simulink library "powerlib2"  (Simulink 6.0)
settings: Solver=ode45  SolverMode=SingleTasking  StartTime=0.0  StopTime=10.0  RelTol=1e-3
undefined symbols (not defined in the file or in its folder): com, ctrl1, Da, DiscIntNeverNeededParam, dtha, etat, FA, gcbh, Ha, Ka, Lm, Ls, powericonV2, q0, Rm, Rs, sel, st_a, st_b, st_c, sta, stb, stc, T1, T2, T3, T4
libraries: powerlib2 x55, simulink_extras x5, powerlib_extras x4, powerlib_modelsV2 x4, simulink x1
(part 4 of 6)

== system powerlib2/Power Electronics ==
  note: ____ D e v i c e s __________________________________________________
  note: ____ E x t r a s ____________________________________________________
  "  Extra Library " : Subsystem
      settings: OpenFcn=sys=sprintf('%s\n%s','powerlib_extras/Discrete ','Control Blocks');powerlib_extras([],[],[],'load');open_system(sys)
      mask Display: disp(['Discrete Control blocks'])
  "  Extra Library 1" : Subsystem
      settings: OpenFcn=sys=sprintf('%s\n%s','powerlib_extras/Control ','Blocks');powerlib_extras([],[],[],'load');open_system(sys)
      mask Display: disp(['Control blocks'])
  Detailed Thyristor : Subsystem  Tag=PoWeRsYsTeMbLoCk  LoadFcn=powericonV2('psblfblk',bdroot,'gotofrom','Load');  mask(Detailed Thyristor){Ron=1e-3, Lon=0, Vf=0.8, IL=0.1, Tq=100e-6, IC=0, Rs=10, Cs=4.7e-6, PSBOutputType=10}
      mask prompts: Ron "Resistance Ron (Ohms) :"; Lon "Inductance Lon (H) :"; Vf "Forward voltage Vf (V) :"; IL "Latching current Il (A) :"; Tq "Turn-off time Tq (s) :"; IC "Initial current Ic (A) :"; Rs "Snubber resistance Rs (Ohms) :"; Cs "Snubber capacitance Cs (F) :"; PSBOutputType "Output type [1=PSB  0=simulink output]"
      mask help:
      | Detailed model of Thyristor in parallel with a series RC snubber circuit. In on-state the Thyristor model  has an internal resistance (Ron) and inductance (Lon).  For most applications the internal inductance should be set to zero. In off-state the Detailed Thyristor  as an impedance.
      |
      | Best accuracy is achieved when Tq is larger than the simulation step size.
      mask init:
      | s=powericonV2('PowerSwitch',Rs,Cs);
      settings: CopyFcn=powericonV2('psblfblk',bdroot,'gotofrom','Copy');
      mask Help: web(psbhelp);
      mask Display: plot(-140,-140,140,140,2*[-30,-30,0,-30,-30,-55]+25,(2*[20,0,20,41,20,20]+8),[0,0]+25,(2*[0,40]+8),2*[37.5,0]+25,(2*[20,20]+8),2*[10,10,0]+25,(1*[-15,6,20]+12),s*[-65,-65,-20,-20,40,40,85,85,85,40,40,-20,-20],s*[48,-20,-20,-10,-10,-20,-20,48,-20,-20,-30,-30,-20])
  Diode : Subsystem  Tag=PoWeRsYsTeMbLoCk  LoadFcn=powericonV2('psblfblk',bdroot,'from','Load');  mask(Diode){Ron=0.01, Lon=0, Vf=0.8, IC=0, Rs=10, Cs=0.01e-6, PSBOutputType=10}
      mask prompts: Ron "Resistance Ron (Ohms) :"; Lon "Inductance Lon (H) :"; Vf "Forward voltage Vf (V) :"; IC "Initial current Ic (A) :"; Rs "Snubber resistance Rs (Ohms) :"; Cs "Snubber capacitance Cs (F) :"; PSBOutputType "Output type [1=PSB  0=simulink output]"
      mask help: Implements a diode in parallel with a series RC snubber circuit. In on-state the Diode model has an internal resistance (Ron) and inductance (Lon). For most applications the internal inductance should be set to zero. The Diode impedance is infinite in off-state mode.
      mask init:
      | s=powericonV2('PowerSwitch',Rs,Cs);
      settings: CopyFcn=powericonV2('psblfblk',bdroot,'from','Copy');
      mask Help: web(psbhelp);
      mask Display: plot(-140,-140,150,140,2*[30,30,59,30,30,0]-75,(2*[71,50,72,92,71,71]-92),2*[59,59]-75,(2*[50,93]-92),[116,59]-16,(2*[71,71]-90),s*[-65,-65,-20,-20,40,40,85,85,85,40,40,-20,-20],s*[52,-20,-20,-10,-10,-20,-20,52,-20,-20,-30,-30,-20])
  Gto : Subsystem  Tag=PoWeRsYsTeMbLoCk  LoadFcn=powericonV2('psblfblk',bdroot,'gotofrom','Load');  mask(Gto){Ron=0.01, Lon=1e-6, Vf=1, Tf=10e-6, Tt=20e-6, IC=0, Rs=10, Cs=0.01e-6, PSBOutputType=10}
      mask prompts: Ron "Resistance Ron (Ohms) :"; Lon "Inductance Lon (H) :"; Vf "Forward voltage Vf (V) :"; Tf "Current 10% fall time Tf (s) :"; Tt "Current tail time Tt (s) :"; IC "Initial current Ic (A) :"; Rs "Snubber resistance Rs (Ohms) :"; Cs "Snubber capacitance Cs (F) :"; PSBOutputType "Output type [1=PSB  0=simulink output]"
      mask help:
      | Implements a GTO thyristor in parallel with a series RC snubber circuit. In on-state the GTO model has internal resistance (Ron) and inductance (Lon). In off-state the GTO model has infinite impedance. The internal inductance cannot be set to zero.
      | Discretization of the GTO is available only through the Universal Bridge block.
      mask init:
      | s=powericonV2('PowerSwitch',Rs,Cs);
      settings: CopyFcn=powericonV2('psblfblk',bdroot,'gotofrom','Copy');
      mask Help: web(psbhelp);
      mask Display: plot(-140,-140,140,140,2*[-30,-30,0,-30,-30,-60]+25,(2*[20,0,20,41,20,20]+8),[0,0]+25,(2*[0,40]+8),2*[35,0]+25,(2*[20,20]+8),2*[10,10,0]+25,(2*[-15,6,20]+8),[20,0]+35,[-8,-8],s*[-75,-75,-20,-20,20,20,75,75,75,20,20,-20,-20],s*([78,0,0,10,10,0,0,78,0,0,-10,-10,0]-30))
  IGBT : Subsystem  Tag=PoWeRsYsTeMbLoCk  LoadFcn=powericonV2('psblfblk',bdroot,'gotofrom','Load');  mask(IGBT){Ron=0.01, Lon=1e-6, Vf=1, Tf=1e-6, Tt=2e-6, IC=0, Rs=0, Cs=0.01e-6, PSBOutputType=10}
      mask prompts: Ron "Resistance Ron (Ohms) :"; Lon "Inductance Lon (H) :"; Vf "Forward voltage Vf (V) :"; Tf "Current 10% fall time Tf (s) :"; Tt "Current tail time Tt (s):"; IC "Initial current Ic (A) :"; Rs "Snubber resistance Rs (Ohms) :"; Cs "Snubber capacitance Cs (F) :"; PSBOutputType "Output type [1=PSB  0=simulink output]"
      mask help:
      | Implements an IGBT device  in parallel with a series RC snubber circuit. In on-state the IGBT model has internal resistance (Ron) and inductance (Lon). In off-state the IGBT model has infinite impedance. The internal inductance cannot be set to zero.
      | Discretization of the IGBT is available only through the Universal Bridge block.
      mask init:
      | s=powericonV2('PowerSwitch',Rs,Cs);
      settings: CopyFcn=powericonV2('psblfblk',bdroot,'gotofrom','Copy');
      mask Help: web(psbhelp);
      mask Display: plot(-15,0,115,100,[82,82,18],[16,35,35],[3,19,35,18,80,60,76,97],[65,65,45,45,45,45,65,65],[81,83,72,81]-7,[65,58,60,65],s*([-75,-75,-20,-20,20,20,75,75,75,20,20,-20,-20]*.45+50),s*([0,50,50,60,60,50,50,0,50,50,40,40,50]*.4+65))
  Ideal Switch : Subsystem  Tag=PoWeRsYsTeMbLoCk  LoadFcn=powericonV2('psblfblk',bdroot,'gotofrom','Load');  mask(Ideal Switch){Ron=0.01, Lon=0, IC=0, Rs=0.1, Cs=0.01e-6, PSBOutputType=10}
      mask prompts: Ron "Internal resistance Ron (Ohms) :"; Lon "Inductance Lon (H) :"; IC "Initial state (0 for 'open', 1 for 'closed') :"; Rs "Snubber resistance Rs (Ohms) :"; Cs "Snubber capacitance Cs (F) :"; PSBOutputType "Output type [1=PSB  0=simulink output]"
      mask help:
      | Switch controlled by a gate signal, in parallel with a series RC snubber circuit. In on-state the Switch model has an internal resistance (Ron) . In off-state this internal resistance is infinite. The internal resistance must be greather than zero.
      |
      | The switch model is on-state when the gate signal (g) is set to 1.
      mask init:
      | s=powericonV2('PowerSwitch',Rs,Cs);
      settings: CopyFcn=powericonV2('psblfblk',bdroot,'gotofrom','Copy');
      mask Help: web(psbhelp);
      mask Display: plot(-140,-140,140,140,[-100,-30,0],[50,50,85],[20,100],[50,50],s*[-75,-75,-20,-20,20,20,75,75,75,20,20,-20,-20],s*[50,0,0,10,10,0,0,50,0,0,-10,-10,0])
  Mosfet : Subsystem  Tag=PoWeRsYsTeMbLoCk  LoadFcn=powericonV2('psblfblk',bdroot,'gotofrom','Load');  mask(Mosfet){Ron=0.001, Lon=1e-6, Rd=.001, IC=0, Rs=10, Cs=0.01e-6, PSBOutputType=10}
      mask prompts: Ron "MOSFET on-state resistance Ron (Ohms) :"; Lon "MOSFET on-state inductance Lon (H) :"; Rd "Internal diode resistance Rd  (Ohms) :"; IC "Initial current Ic (A) :"; Rs "Snubber resistance Rs (Ohms) :"; Cs "Snubber capacitance Cs (F) :"; PSBOutputType "Output type [1=PSB  0=simulink output]"
      mask help:
      | MOSFET in parallel with a series RC snubber circuit. In on-state the MOSFET model has internal resistance (Ron) and inductance (Lon). In off-state the MOSFET model has infinite impedance. The internal inductance cannot be set to zero.
      | Discretization of the MOSFET is available only through the Universal Bridge block.
      mask init:
      | s=powericonV2('PowerSwitch',Rs,Cs);
      settings: CopyFcn=powericonV2('psblfblk',bdroot,'gotofrom','Copy');
      mask Help: web(psbhelp);
      mask Display: plot(-160,-140,140,140,2*[33,23,28,28,10,10,35,55,55,90,55,55,35,35,35,35,0]-100,(2*[28,28,28,50,50,75,75,65,75,75,75,85,75,65,85,75,75]-100),2*[50,39,45,38,52,45,45,65,65,60,70,65,65,82,82]-100,(2*[28,28,28,39,39,28,50,50,28,28,28,28,50,50,75]-100),2*[70,70,23]-100,(2*[7,20,20]-100),s*[-50,-50,-30,-30,10,10,32,32,32,10,10,-30,-30],s*([45,80,80,85,85,80,80,45,80,80,75,75,80]+5))
  Three-Level Bridge : Subsystem  Tag=PoWeRsYsTeMbLoCk  LoadFcn=powericonV2('psblfblk',bdroot,'configurable bridge','Copy')  mask(Three-Level Bridge){arms=3, confi=ABC as input terminals, Rs=1e5, Cs=inf, device=GTO / Diodes, Ron=1e-3, PAr_vf=[  0  0  ], mesure=None, PSBOutputType=111}
      mask prompts: arms "Number of bridge arms:"; confi "Port configuration"; Rs "Snubber resistance Rs (Ohms)"; Cs "Snubber capacitance Cs (F)"; device "Power Electronic device"; Ron "Internal resistance Ron (Ohms)"; PAr_vf "Forward voltages  [ Device Vf(V) , Diode Vfd(V)]"; mesure "Measurements"; PSBOutputType "Output type [1=PSB  0=simulink output]"
      mask help: This block implements a three-level bridge of selected forced-commutated power electronics devices. Series RC snubber circuits are connected in parallel with each switch device.
      mask init:
      | if device==4
      |     switch arms
      |     case 1
      |         selection1 = [1,2,4];
      |         selection2 = [1,3,4];
      |     case 2
      |         selection1 = [1,2,4,5,6,8];
      |         selection2 = [1,3,4,5,7,8];
      |     case 3
      |         selection1 = [1,2,4,5,6,8,9,10,12];
      |         selection2 = [1,3,4,5,7,8,9,11,12];
      |     end
      | else
      |     selection1 = [1:4*arms];
      |     selection2 = [1:4*arms];
      | end
      | 
      | powericonV2('psbcb6thy',gcb,'Three-level device configuration');
      | powericonV2('psbcb6thy',gcb,'3Level port configuration');
      settings: CopyFcn=powericonV2('psblfblk',bdroot,'configurable bridge','Copy')
      mask Help: web(psbhelp);
      mask StyleString: popup(1|2|3),popup(ABC as input terminals|ABC as output terminals),edit,edit,popup(GTO / Diodes|MOSFET / Diodes|IGBT / Diodes|Ideal Switches),edit,edit,popup(None|All device currents|Phase-to-Neutral and DC voltages|All voltages and currents),edit
      mask CallbackString: powericonV2('psbcb6thy',gcb,'3Level port configuration')|powericonV2('psbcb6thy',gcb,'3Level port configuration')|||powericon('psbcb6thy',gcb,'Three-level device configuration')||||
      mask Display: plot(0,0,100,100,[40 28 52 40 24 52 40 40],[40 60 60 40 40 40 40 10],[40,40],[90,60],[16 28 40],[25,25,40],[21.6 35.2],[25,40],[65 57 73 65 57 73 65 65],[54 42 42 54 54 54 54 66],[40 65 65],[24 24 42],[65 65 40],[66,76,76]);
  Thyristor : Subsystem  Tag=PoWeRsYsTeMbLoCk  LoadFcn=powericonV2('psblfblk',bdroot,'gotofrom','Load');  mask(Thyristor){Ron=1e-03, Lon=0, Vf=0.8, IC=0, Rs=10, Cs=4.7e-6, PSBOutputType=10}
      mask prompts: Ron "Resistance Ron (Ohms) :"; Lon "Inductance Lon (H) :"; Vf "Forward voltage Vf (V) :"; IC "Initial current Ic (A) :"; Rs "Snubber resistance Rs (Ohms) :"; Cs "Snubber capacitance Cs (F) :"; PSBOutputType "Output type [1=PSB  0=simulink output]"
      mask help: Thyristor in parallel with a series RC snubber circuit. In on-state the Thyristor model has an internal resistance (Ron) and inductance (Lon). For most applications the internal inductance should be set to zero. In off-state the Thyristor as an infinite impedance.
      mask init:
      | s=powericonV2('PowerSwitch',Rs,Cs);
      settings: CopyFcn=powericonV2('psblfblk',bdroot,'gotofrom','Copy');
      mask Help: web(psbhelp);
      mask Display: plot(-140,-140,140,140,2*[-30,-30,0,-30,-30,-55]+25,(2*[20,0,20,41,20,20]+8),[0,0]+25,(2*[0,40]+8),2*[37.5,0]+25,(2*[20,20]+8),2*[10,10,0]+25,(1*[-15,6,20]+12),s*[-65,-65,-20,-20,40,40,85,85,85,40,40,-20,-20],s*[48,-20,-20,-10,-10,-20,-20,48,-20,-20,-30,-30,-20])
  Universal Bridge : Subsystem  Tag=PoWeRsYsTeMbLoCk  LoadFcn=powericonV2('psblfblk',bdroot,'configurable bridge','Copy')  mask(Universal Bridge){arms=3, confi=ABC as input terminals, injcc=1e5, cf=inf, device=Thyristors, Ron=1e-3, Lon=0, VFs=[  0  0  ], Vf=0, gtoparameters=[ 10e-6 , 20e-6 ], igbtparameters=[ 1e-6 , 2e-6 ], mesure=None, PSBOutputType=111}
      mask prompts: arms "Number of bridge arms:"; confi "Port configuration"; injcc "Snubber resistance Rs (Ohms)"; cf "Snubber capacitance Cs (F)"; device "Power Electronic device"; Ron "Ron (Ohms)"; Lon "Lon (H)"; VFs "Forward voltages  [ Device Vf(V) , Diode Vfd(V)]"; Vf "Forward voltage Vf (V)"; gtoparameters "[  Tf (s) , Tt (s)  ]"; igbtparameters "[  Tf (s) , Tt (s)  ]"; mesure "Measurements"; PSBOutputType "Output type [1=PSB  0=simulink output]"
      mask help: This block implement a bridge of selected power electronics devices. Series RC snubber circuits are connected in parallel with each switch device. For most applications the internal inductance should be set to zero.
      mask init:
      | powericonV2('psbcb6thy',gcb,'device configuration');
      | powericonV2('psbcb6thy',gcb,'port configuration');
      settings: CopyFcn=powericonV2('psblfblk',bdroot,'configurable bridge','Copy')
      mask Help: web(psbhelp);
      mask StyleString: popup(1|2|3),popup(ABC as input terminals|ABC as output terminals),edit,edit,popup(Diodes|Thyristors|GTO / Diodes|MOSFET / Diodes|IGBT / Diodes|Ideal Switches),edit,edit,edit,edit,edit,edit,popup(None|Device voltages|Device currents|UAB UBC UCA UDC voltages|All voltages and currents),edit
      mask CallbackString: powericonV2('psbcb6thy',gcb,'port configuration')|powericonV2('psbcb6thy',gcb,'port configuration')|||powericonV2('psbcb6thy',gcb,'device configuration')||||||||
      mask Display: plot(0,0,100,100,[50,30,70,50,30,70,50,50],[60,30,30,60,60,60,60,90],[50,50],[10,30],[20,35,50],[75,75,60]);

== system powerlib2/powergui ==
  Subsystem : Subsystem

== system powerlib2/Connectors/Bus Bar (horiz) ==
  in_1 : Inport  Port=1  LatchInput=off
  in_2 : Inport  Port=2  LatchInput=off
  g1 : Constant
  t1 : Terminator
  t2 : Terminator
  out_1 : Outport  InitialOutput=0
  wires:
  g1/1 -> out_1/1
  in_1/1 -> t1/1
  in_2/1 -> t2/1

== system powerlib2/Connectors/Bus Bar (thin horiz) ==
  in_1 : Inport  Port=1  LatchInput=off
  in_2 : Inport  Port=2  LatchInput=off
  g1 : Constant
  t1 : Terminator
  t2 : Terminator
  out_1 : Outport  InitialOutput=0
  wires:
  in_2/1 -> t2/1
  in_1/1 -> t1/1
  g1/1 -> out_1/1

== system powerlib2/Connectors/Bus Bar (thin vert) ==
  in_1 : Inport  Port=1  LatchInput=off
  in_2 : Inport  Port=2  LatchInput=off
  g1 : Constant
  g2 : Constant
  t1 : Terminator
  t2 : Terminator
  out_1 : Outport  InitialOutput=0
  out_2 : Outport  Port=2
  wires:
  g1/1 -> out_1/1
  in_1/1 -> t1/1
  in_2/1 -> t2/1
  g2/1 -> out_2/1

== system powerlib2/Connectors/Bus Bar (vert) ==
  in_1 : Inport  Port=1  LatchInput=off
  in_2 : Inport  Port=2  LatchInput=off
  in_3 : Inport  Port=3  LatchInput=off
  g1 : Constant
  g2 : Constant
  t1 : Terminator
  t2 : Terminator
  t3 : Terminator
  out_1 : Outport  InitialOutput=0
  out_2 : Outport  Port=2  InitialOutput=0
  wires:
  g2/1 -> out_2/1
  in_3/1 -> t3/1
  in_2/1 -> t2/1
  in_1/1 -> t1/1
  g1/1 -> out_1/1

== system powerlib2/Connectors/Ground (input) ==
  In_1 : Inport  Port=1  LatchInput=off
  Terminator : Terminator
  wires:
  In_1/1 -> Terminator/1

== system powerlib2/Connectors/Ground (output) ==
  Constant : Constant
  out : Outport  InitialOutput=0
  wires:
  Constant/1 -> out/1

== system powerlib2/Connectors/L connector ==
  In : Inport  Port=1  LatchInput=off
  Enable : EnablePort
  Terminator : Terminator
  wires:
  In/1 -> Terminator/1

== system powerlib2/Connectors/Neutral (input) ==
  In_1 : Inport  Port=1  LatchInput=off
  Terminator : Terminator
  wires:
  In_1/1 -> Terminator/1

== system powerlib2/Connectors/Neutral (output) ==
  Constant : Constant
  Outport : Outport  InitialOutput=0
  wires:
  Constant/1 -> Outport/1

== system powerlib2/Connectors/T connector ==
  In : Inport  Port=1  LatchInput=off
  Enable : EnablePort
  Ground : Ground
  Terminator : Terminator
  Out : Outport  InitialOutput=0
  wires:
  In/1 -> Terminator/1
  Ground/1 -> Out/1

== system powerlib2/Electrical Sources/3-Phase  Programmable  Voltage Source ==
  note: Pierre Giroux, Gilbert Sybille
      | Power System Laboratory, IREQ
      | Hydro-Quebec
  note: Programmable 3-phase Voltage Source
  N : Inport  Orientation=left  Port=1  LatchInput=off
  Bus Bar1 : powerlib2/Connectors/Bus Bar (horiz)  Tag=PoWeRsYsTeMbLoCk  Orientation=down  entrees=4  sorties=0  PSBOutputType=1111111111111111111111111111111111111111111111111111111111111111111111111
  Controlled Voltage Source1 : powerlib2/Electrical Sources/Controlled Voltage Source  Tag=PoWeRsYsTeMbLoCk  Description=source block  initsrc=on  srctyp=AC  iv=Par_Vps(1)  iph=Par_Vps(2)  ifreq=Par_Vps(3)  mesure=None  PSBOutputType=11
  Controlled Voltage Source2 : powerlib2/Electrical Sources/Controlled Voltage Source  Tag=PoWeRsYsTeMbLoCk  Description=source block  initsrc=on  srctyp=AC  iv=Par_Vps(1)  iph=Par_Vps(2)-120  ifreq=Par_Vps(3)  mesure=None  PSBOutputType=11
  Controlled Voltage Source3 : powerlib2/Electrical Sources/Controlled Voltage Source  Tag=PoWeRsYsTeMbLoCk  Description=source block  initsrc=on  srctyp=AC  iv=Par_Vps(1)  iph=Par_Vps(2)+120  ifreq=Par_Vps(3)  mesure=None  PSBOutputType=11
  Demux : Demux  Outputs=3
  Source : Subsystem  mask(Discrete 3-phase Programmable Source){Par_Vps=Par_Vps, VariationEntity=VariationEntity, VariationType=VariationType, VariationStep=VariationStep, VariationRate=VariationRate, VariationMag=VariationMag, VariationFreq=VariationFreq, Par_Timing_Variation=Par_Timing_Variation, SinglePhase=SinglePhase, Yampli=Yampli, Xtime=Xtime, HarmonicGeneration=HarmonicGeneration, Par_HarmoA=Par_HarmoA, Par_HarmoB=Par_HarmoB, Par_Timing_Harmo=Par_Timing_Harmo, Ts=evalin('base','Ts')}
      mask prompts: Par_Vps "Positive-sequence: [ Amplitude  Phase(degrees)   Freq. (Hz) ]"; VariationEntity "Time variation of:"; VariationType "Type of variation:"; VariationStep "Step magnitude:"; VariationRate "Rate of change (value/s):"; VariationMag "Amplitude of the modulation:"; VariationFreq "Frequency of the modulation(Hz):"; Par_Timing_Variation "Variation timing (s) : [ Start   End ]"; SinglePhase "1-phase only"; Yampli "Amplitude values:"; Xtime "Time values:"; HarmonicGeneration "Harmonic generation:"; Par_HarmoA "A:  [ Order(n)   Amplitude  Phase(degrees)  Seq(0, 1 or 2) ]"; Par_HarmoB "B:  [ Order(n)   Amplitude  Phase(degrees)  Seq(0, 1 or 2) ]"; Par_Timing_Harmo "Harmonic timing (s) : [ Start   End ]"; Ts "Sample time:"
      mask help: Use this discrete block to generate a set of three-phase sinusoidal voltages or currents a, b and c. Time variation for the amplitude, phase and frequency of the fundamental can be pre-programmed. In addition, two harmonics can be surimposed on the fundamental.
      mask init:
      | Mag_Vps=Par_Vps(1);
      | Phase_Vps=Par_Vps(2);
      | Freq_Vps=Par_Vps(3);
      | Ton_Variation=Par_Timing_Variation(1);
      | Toff_Variation=Par_Timing_Variation(2);
      | n_HarmoA=Par_HarmoA(1);
      | Mag_HarmoA=Par_HarmoA(2);
      | Phase_HarmoA=Par_HarmoA(3);
      | Seq_HarmoA=Par_HarmoA(4);
      | if n_HarmoA==0
      |     Phase_HarmoA=90;
      |     Seq_HarmoA=0;
      | end
      | n_HarmoB=Par_HarmoB(1);
      | Mag_HarmoB=Par_HarmoB(2);
      | Phase_HarmoB=Par_HarmoB(3);
      | Seq_HarmoB=Par_HarmoB(4);
      | if n_HarmoB==0
      |     Phase_HarmoB=90;
      |     Seq_HarmoB=0;
      | end
      | Ton_Harmo=Par_Timing_Harmo(1);
      | Toff_Harmo=Par_Timing_Harmo(2);
      | if length(Yampli) ~= length(Xtime),
      |    h=errordlg(' The vectors specifying the time and amplitude pairs must have the same length ' , 'Parameter error');
      | end
      | if Xtime(1)~=0,
      |    h=errordlg(' A pair time-amplitude must be specified at time zero' , 'Parameter error');
      | Xtime=[0 Xtime];
      | Yampli=[0 Yampli];
      | end
      | n=length(Xtime); vec_dt= [Xtime,0] - [0,Xtime] ; vec_dt=vec_dt(2:n);
      | if any(vec_dt<=0)
      |    h=errordlg(' All transition times must be in increasing order' , 'Parameter error');
      | end
      mask CallbackString: |parametres=get_param(gcb,'MaskValues');p2=parametres{2};p3=parametres{3};p12=parametres{12};if strcmp(p3,'Step');param4='on';param5='off';param6='off';param7='off';param8='on';param9='off';param10='off';param11='off';elseif strcmp(p3,'Ramp');param4='off';param5='on';param6='off';param7='off';param8='on';param9='off';param10='off';param11='off';elseif strcmp(p3,'Modulation');param4='off';param5='off';param6='on';param7='on';param8='on';param9='off';param10='off';param11='off';else;param4='off';param5='off';param6='off';param7='off';param8='off';param9='on';param10='on';param11='on';end;if strcmp(p2,'None');param3='off';param4='off';param5='off';param6='off';param7='off';param8='off';param9='off';param10='off';param11='off';else;param3='on';end;if strcmp(p12,'on');param13='on';param14='on';param15='on';else;param13='off';param14='off';param15='off';end;visible={'on','on',param3,param4,param5,param6,param7,param8,param9,param10,param11,'on',param13,param14,param15,'on'};set_param(gcb,'MaskVisibilities',visible)|parametres=get_param(gcb,'MaskValues');p2=parametres{2};p3=parametres{3};p12=parametres{12};if strcmp(p3,'Step');param4='on';param5='off';param6='off';param7='off';param8='on';param9='off';param10='off';param11='off';elseif strcmp(p3,'Ramp');param4='off';param5='on';param6='off';param7='off';param8='on';param9='off';param10='off';param11='off';elseif strcmp(p3,'Modulation');param4='off';param5='off';param6='on';param7='on';param8='on';param9='off';param10='off';param11='off';else;param4='off';param5='off';param6='off';param7='off';param8='off';param9='on';param10='on';param11='on';end;if strcmp(p2,'None');param3='off';param4='off';param5='off';param6='off';param7='off';param8='off';param9='off';param10='off';param11='off';else;param3='on';end;if strcmp(p12,'on');param13='on';param14='on';param15='on';else;param13='off';param14='off';param15='off';end;visible={'on','on',param3,param4,param5,param6,param7,param8,param9,param10,param11,'on',param13,param14,param15,'on'};set_param(gcb,'MaskVisibilities',visible)|||||||||parametres=get_param(gcb,'MaskValues');p2=parametres{2};p3=parametres{3};p12=parametres{12};if strcmp(p3,'Step');param4='on';param5='off';param6='off';param7='off';param8='on';param9='off';param10='off';param11='off';elseif strcmp(p3,'Ramp');param4='off';param5='on';param6='off';param7='off';param8='on';param9='off';param10='off';param11='off';elseif strcmp(p3,'Modulation');param4='off';param5='off';param6='on';param7='on';param8='on';param9='off';param10='off';param11='off';else;param4='off';param5='off';param6='off';param7='off';param8='off';param9='on';param10='on';param11='on';end;if strcmp(p2,'None');param3='off';param4='off';param5='off';param6='off';param7='off';param8='off';param9='off';param10='off';param11='off';else;param3='on';end;if strcmp(p12,'on');param13='on';param14='on';param15='on';else;param13='off';param14='off';param15='off';end;visible={'on','on',param3,param4,param5,param6,param7,param8,param9,param10,param11,'on',param13,param14,param15,'on'};set_param(gcb,'MaskVisibilities',visible)||||
  A : Outport
  B : Outport  Port=2
  C : Outport  Port=3
  wires:
  N/1 -> Bus Bar1/4
  Demux/3 -> Controlled Voltage Source3/1
  Demux/2 -> Controlled Voltage Source2/1
  Demux/1 -> Controlled Voltage Source1/1
  Source/1(abc) -> Demux/1
  Controlled Voltage Source3/2 -> Bus Bar1/3
  Controlled Voltage Source2/2 -> Bus Bar1/2
  Controlled Voltage Source1/2 -> Bus Bar1/1
  Controlled Voltage Source3/1 -> C/1
  Controlled Voltage Source2/1 -> B/1
  Controlled Voltage Source1/1 -> A/1

== system powerlib2/Electrical Sources/3-Phase Source ==
  N : Inport  Port=1  LatchInput=off
  Constant1 : Constant  Value=NaN
  Constant2 : Constant  Value=NaN
  Constant3 : Constant  Value=NaN
  Terminator : Terminator
  A : Outport
  B : Outport  Port=2
  C : Outport  Port=3
  wires:
  N/1 -> Terminator/1
  Constant2/1 -> A/1
  Constant1/1 -> B/1
  Constant3/1 -> C/1

== system powerlib2/Electrical Sources/AC Current Source ==
  in_1 : Inport  Port=1  LatchInput=off
  Constant : Constant  Value=complex(A*cos(P*pi/180),A*sin(P*pi/180))
  Constant1 : Constant  Value=NaN
  Mux : Mux  Inputs=2
  Sine Wave : Sin  Amplitude=A  Frequency=2*pi*F  Phase=P*pi/180  SampleTime=stime
  Terminator : Terminator
  out_1 : Outport  InitialOutput=0
  tag scope: tp200416=global
  wires:
  in_1/1 -> Terminator/1
  Constant1/1 -> out_1/1
  Sine Wave/1 -> Mux/1
  Constant/1 -> Mux/2
  Mux/1 -> [tp200416]

== system powerlib2/Electrical Sources/AC Voltage Source ==
  in_1 : Inport  Port=1  LatchInput=off
  Constant : Constant  Value=complex(A*cos(P*pi/180),A*sin(P*pi/180))
  Constant1 : Constant  Value=NaN
  Mux : Mux  Inputs=2
  Sine Wave : Sin  Amplitude=A  Frequency=2*pi*F  Phase=P*pi/180  SampleTime=stime
  Terminator : Terminator
  out_1 : Outport  InitialOutput=0
  tag scope: tp200422=global
  wires:
  Constant/1 -> Mux/2
  in_1/1 -> Terminator/1
  Constant1/1 -> out_1/1
  Sine Wave/1 -> Mux/1
  Mux/1 -> [tp200422]

== system powerlib2/Electrical Sources/Controlled Current Source ==
  signal : Inport  Port=1  LatchInput=off
  Constant2 : Constant  Value=NaN
  Constant3 : Constant  Value=NaN
  Mux : Mux  Inputs=2
  " " : Outport  InitialOutput=0
  "  " : Outport  Port=2  InitialOutput=0
  tag scope: tp200426=global
  wires:
  Constant2/1 -> " "/1
  Constant3/1 -> "  "/1
  Mux/1 -> [tp200426]
  signal/1 -> Mux/1, Mux/2

== system powerlib2/Electrical Sources/Controlled Voltage Source ==
  signal : Inport  Port=1  LatchInput=off
  Constant1 : Constant  Value=NaN
  Constant2 : Constant  Value=NaN
  Mux : Mux  Inputs=2
  + : Outport  InitialOutput=0
  - : Outport  Port=2  InitialOutput=0
  tag scope: tp200433=global
  wires:
  Constant1/1 -> +/1
  Constant2/1 -> -/1
  signal/1 -> Mux/1, Mux/2
  Mux/1 -> [tp200433]

== system powerlib2/Electrical Sources/DC Voltage Source ==
  in_1 : Inport  Port=1  LatchInput=off
  Constant : Constant  Value=complex(V,0)
  Constant1 : Constant  Value=NaN
  Constant2 : Constant  Value=V
  Mux : Mux  Inputs=2
  Terminator : Terminator
  out_1 : Outport  InitialOutput=0
  tag scope: tp200438=global
  wires:
  Constant1/1 -> out_1/1
  in_1/1 -> Terminator/1
  Mux/1 -> [tp200438]
  Constant2/1 -> Mux/1
  Constant/1 -> Mux/2

== system powerlib2/Elements/3-Phase Dynamic Load ==
  A : Inport  Port=1  LatchInput=off
  B : Inport  Port=2  LatchInput=off
  C : Inport  Port=3  LatchInput=off
  PQ : Ground
  Terminator1 : Terminator
  Terminator2 : Terminator
  Terminator4 : Terminator
  m : Outport
  tag scope: tp200444=global
  wires:
  A/1 -> Terminator1/1
  B/1 -> Terminator2/1
  C/1 -> Terminator4/1
  PQ/1 -> [tp200444]
  [tp200449] -> m/1

== system powerlib2/Elements/3-Phase Mutual Inductance Z1-Z0 ==
  A : Inport  Port=1  LatchInput=off
  B : Inport  Port=2  LatchInput=off
  C : Inport  Port=3  LatchInput=off
  Mutual Inductance : powerlib2/Elements/Mutual Inductance  Tag=PoWeRsYsTeMbLoCk  a=[Rs Ls]  b=[Rs Ls]  w3check=on  c=[Rs Ls]  d=[Rm Lm]  mesure=None  PSBOutputType=111
  " A" : Outport  InitialOutput=0
  " B" : Outport  Port=2  InitialOutput=0
  " C" : Outport  Port=3  InitialOutput=0
  wires:
  Mutual Inductance/1 -> " A"/1
  Mutual Inductance/2 -> " B"/1
  Mutual Inductance/3 -> " C"/1
  C/1 -> Mutual Inductance/3
  B/1 -> Mutual Inductance/2
  A/1 -> Mutual Inductance/1

== system powerlib2/Elements/3-Phase Parallel RLC Branch ==
  A : Inport  Port=1  LatchInput=off
  B : Inport  Port=2  LatchInput=off
  C : Inport  Port=3  LatchInput=off
  Parallel RLC Branch 1 : powerlib2/Elements/Parallel RLC Branch  Tag=PoWeRsYsTeMbLoCk  a=R  b=L  c=C  mesure=None  PSBOutputType=1
  Parallel RLC Branch 2 : powerlib2/Elements/Parallel RLC Branch  Tag=PoWeRsYsTeMbLoCk  a=R  b=L  c=C  mesure=None  PSBOutputType=1
  Parallel RLC Branch 3 : powerlib2/Elements/Parallel RLC Branch  Tag=PoWeRsYsTeMbLoCk  a=R  b=L  c=C  mesure=None  PSBOutputType=1
  " A" : Outport  InitialOutput=0
  " B" : Outport  Port=2  InitialOutput=0
  " C" : Outport  Port=3  InitialOutput=0
  wires:
  Parallel RLC Branch 1/1 -> " A"/1
  A/1 -> Parallel RLC Branch 1/1
  Parallel RLC Branch 2/1 -> " B"/1
  B/1 -> Parallel RLC Branch 2/1
  Parallel RLC Branch 3/1 -> " C"/1
  C/1 -> Parallel RLC Branch 3/1

== system powerlib2/Elements/3-Phase Parallel RLC Load ==
  A : Inport  Port=1  LatchInput=off
  B : Inport  Port=2  LatchInput=off
  C : Inport  Port=3  LatchInput=off
  Ground (input) : powerlib2/Connectors/Ground (input)  Tag=PoWeRsYsTeMbLoCk  Orientation=down
  Ground (input)1 : powerlib2/Connectors/Ground (input)  Tag=PoWeRsYsTeMbLoCk  Orientation=down
  Ground (input)2 : powerlib2/Connectors/Ground (input)  Tag=PoWeRsYsTeMbLoCk  Orientation=down
  Parallel RLC Load 1 : powerlib2/Elements/Parallel RLC Load  Tag=PoWeRsYsTeMbLoCk  a=Vpp/sqrt(3)  b=fn  c=P3/3  d=QL3/3  e=QC3/3  mesure=None  PSBOutputType=1
  Parallel RLC Load 2 : powerlib2/Elements/Parallel RLC Load  Tag=PoWeRsYsTeMbLoCk  a=Vpp/sqrt(3)  b=fn  c=P3/3  d=QL3/3  e=QC3/3  mesure=None  PSBOutputType=1
  Parallel RLC Load 3 : powerlib2/Elements/Parallel RLC Load  Tag=PoWeRsYsTeMbLoCk  a=Vpp/sqrt(3)  b=fn  c=P3/3  d=QL3/3  e=QC3/3  mesure=None  PSBOutputType=1
  wires:
  Parallel RLC Load 1/1 -> Ground (input)/1
  A/1 -> Parallel RLC Load 1/1
  Parallel RLC Load 2/1 -> Ground (input)1/1
  B/1 -> Parallel RLC Load 2/1
  Parallel RLC Load 3/1 -> Ground (input)2/1
  C/1 -> Parallel RLC Load 3/1

== system powerlib2/Elements/3-Phase Series RLC Branch  ==
  A : Inport  Port=1  LatchInput=off
  B : Inport  Port=2  LatchInput=off
  C : Inport  Port=3  LatchInput=off
  Series RLC Branch 1 : powerlib2/Elements/Series RLC Branch  Tag=PoWeRsYsTeMbLoCk  a=R  b=L  c=C  mesure=None  PSBOutputType=1
  Series RLC Branch 2 : powerlib2/Elements/Series RLC Branch  Tag=PoWeRsYsTeMbLoCk  a=R  b=L  c=C  mesure=None  PSBOutputType=1
  Series RLC Branch 3 : powerlib2/Elements/Series RLC Branch  Tag=PoWeRsYsTeMbLoCk  a=R  b=L  c=C  mesure=None  PSBOutputType=1
  "A " : Outport  InitialOutput=0
  "B " : Outport  Port=2  InitialOutput=0
  "C " : Outport  Port=3  InitialOutput=0
  wires:
  A/1 -> Series RLC Branch 1/1
  Series RLC Branch 1/1 -> "A "/1
  B/1 -> Series RLC Branch 2/1
  Series RLC Branch 2/1 -> "B "/1
  C/1 -> Series RLC Branch 3/1
  Series RLC Branch 3/1 -> "C "/1

== system powerlib2/Elements/3-Phase Series RLC Load ==
  A : Inport  Port=1  LatchInput=off
  B : Inport  Port=2  LatchInput=off
  C : Inport  Port=3  LatchInput=off
  Ground3 : powerlib2/Connectors/Ground (input)  Tag=PoWeRsYsTeMbLoCk  Orientation=down
  Ground4 : powerlib2/Connectors/Ground (input)  Tag=PoWeRsYsTeMbLoCk  Orientation=down
  Ground5 : powerlib2/Connectors/Ground (input)  Tag=PoWeRsYsTeMbLoCk  Orientation=down
  RLC 1 : powerlib2/Elements/Series RLC Load  Tag=PoWeRsYsTeMbLoCk  a=Vpp/sqrt(3)  b=fn  c=P3/3  d=QL3/3  e=QC3/3  mesure=None  PSBOutputType=1
  RLC 2 : powerlib2/Elements/Series RLC Load  Tag=PoWeRsYsTeMbLoCk  a=Vpp/sqrt(3)  b=fn  c=P3/3  d=QL3/3  e=QC3/3  mesure=None  PSBOutputType=1
  RLC 3 : powerlib2/Elements/Series RLC Load  Tag=PoWeRsYsTeMbLoCk  a=Vpp/sqrt(3)  b=fn  c=P3/3  d=QL3/3  e=QC3/3  mesure=None  PSBOutputType=1
  wires:
  RLC 1/1 -> Ground5/1
  A/1 -> RLC 1/1
  RLC 2/1 -> Ground4/1
  B/1 -> RLC 2/1
  RLC 3/1 -> Ground3/1
  C/1 -> RLC 3/1

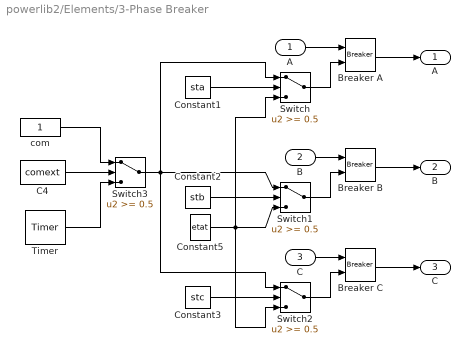
== system powerlib2/Elements/3-Phase Breaker ==
  A : Inport  Port=1  LatchInput=off
  B : Inport  Port=2  LatchInput=off
  C : Inport  Port=3  LatchInput=off
  Breaker A : powerlib2/Elements/Breaker  Tag=PoWeRsYsTeMbLoCk  a=Ron  c=etat  rs=Rp  cs=Cp  times="[ 4/60  5/60 ]"  Ts=0  comext=on  mesure=None  PSBOutputType=1
  Breaker B : powerlib2/Elements/Breaker  Tag=PoWeRsYsTeMbLoCk  a=Ron  c=etat  rs=Rp  cs=Cp  times="[ 4/60  5/60 ]"  Ts=0  comext=on  mesure=None  PSBOutputType=1
  Breaker C : powerlib2/Elements/Breaker  Tag=PoWeRsYsTeMbLoCk  a=Ron  c=etat  rs=Rp  cs=Cp  times="[ 4/60  5/60 ]"  Ts=0  comext=on  mesure=None  PSBOutputType=1
  C4 : Constant  Value=comext
  Constant1 : Constant  Value=sta
  Constant2 : Constant  Value=stb
  Constant3 : Constant  Value=stc
  Constant5 : Constant  Value=etat
  Switch{,1..3} (4 alike) : Switch  Threshold=0.5  InputSameDT=on
  Timer : powerlib_extras/Control  Blocks/Timer  t=sw_times  e=switchings
  com : Constant
  "A " : Outport
  "B " : Outport  Port=2
  "C " : Outport  Port=3
  wires:
  Timer/1 -> Switch3/3
  com/1 -> Switch3/1
  C4/1 -> Switch3/2
  Constant5/1 -> Switch2/3, Switch/3, Switch1/3
  Switch1/1 -> Breaker B/2
  Constant2/1 -> Switch1/2
  Switch2/1 -> Breaker C/2
  Constant3/1 -> Switch2/2
  Switch/1 -> Breaker A/2
  Constant1/1 -> Switch/2
  Breaker C/1 -> "C "/1
  Breaker B/1 -> "B "/1
  Breaker A/1 -> "A "/1
  C/1 -> Breaker C/1
  B/1 -> Breaker B/1
  A/1 -> Breaker A/1
  Switch3/1 -> Switch2/1, Switch/1, Switch1/1

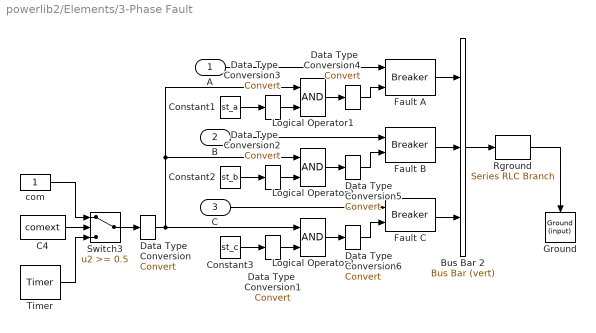
== system powerlib2/Elements/3-Phase Fault ==
  A : Inport  Port=1  LatchInput=off
  B : Inport  Port=2  LatchInput=off
  C : Inport  Port=3  LatchInput=off
  Bus Bar 2 : powerlib2/Connectors/Bus Bar (vert)  Tag=PoWeRsYsTeMbLoCk  entrees=3  sorties=1  PSBOutputType=11111111111111111111111111111111111111111111111111111111111111111111111111111111111111111
  C4 : Constant  Value=comext
  Constant1 : Constant  Value=st_a
  Constant2 : Constant  Value=st_b
  Constant3 : Constant  Value=st_c
  Data Type  Conversion{,1..3} (4 alike) : DataTypeConversion  OutDataTypeMode=boolean  SaturateOnIntegerOverflow=on  RndMeth=Zero
  Data Type  Conversion4 : DataTypeConversion  OutDataTypeMode=double  SaturateOnIntegerOverflow=on  RndMeth=Zero
  Data Type  Conversion5 : DataTypeConversion  OutDataTypeMode=double  SaturateOnIntegerOverflow=on  RndMeth=Zero
  Data Type  Conversion6 : DataTypeConversion  OutDataTypeMode=double  SaturateOnIntegerOverflow=on  RndMeth=Zero
  Fault A : powerlib2/Elements/Breaker  Tag=PoWeRsYsTeMbLoCk  a=Rdef  c=init_a  rs=Rp  cs=Cp  times="[ 4/60  5/60 ]"  Ts=0  comext=on  mesure=None  PSBOutputType=1
  Fault B : powerlib2/Elements/Breaker  Tag=PoWeRsYsTeMbLoCk  a=Rdef  c=init_b  rs=Rp  cs=Cp  times="[ 4/60  5/60 ]"  Ts=0  comext=on  mesure=None  PSBOutputType=1
  Fault C : powerlib2/Elements/Breaker  Tag=PoWeRsYsTeMbLoCk  a=Rdef  c=init_c  rs=Rp  cs=Cp  times="[ 4/60  5/60 ]"  Ts=0  comext=on  mesure=None  PSBOutputType=1
  Ground : powerlib2/Connectors/Ground (input)  Tag=PoWeRsYsTeMbLoCk  Orientation=down
  Logical Operator1 : Logic
  Logical Operator2 : Logic
  Logical Operator3 : Logic
  Rground : powerlib2/Elements/Series RLC Branch  Tag=PoWeRsYsTeMbLoCk  a=Rground  b=0  c=inf  mesure=None  PSBOutputType=1
  Switch3 : Switch  Threshold=0.5  InputSameDT=on
  Timer : powerlib_extras/Control  Blocks/Timer  t=sw_times  e=sw_status
  com : Constant
  wires:
  Data Type  Conversion6/1 -> Fault C/2
  Logical Operator3/1 -> Data Type  Conversion6/1
  Data Type  Conversion5/1 -> Fault B/2
  Logical Operator2/1 -> Data Type  Conversion5/1
  Data Type  Conversion4/1 -> Fault A/2
  Logical Operator1/1 -> Data Type  Conversion4/1
  Data Type  Conversion3/1 -> Logical Operator1/2
  Constant1/1 -> Data Type  Conversion3/1
  Data Type  Conversion2/1 -> Logical Operator2/2
  Constant2/1 -> Data Type  Conversion2/1
  Data Type  Conversion1/1 -> Logical Operator3/2
  Constant3/1 -> Data Type  Conversion1/1
  Data Type  Conversion/1 -> Logical Operator1/1, Logical Operator2/1, Logical Operator3/1
  Switch3/1 -> Data Type  Conversion/1
  Bus Bar 2/1 -> Rground/1
  Rground/1 -> Ground/1
  C/1 -> Fault C/1
  B/1 -> Fault B/1
  Fault B/1 -> Bus Bar 2/2
  Fault C/1 -> Bus Bar 2/3
  A/1 -> Fault A/1
  Fault A/1 -> Bus Bar 2/1
  C4/1 -> Switch3/2
  Timer/1 -> Switch3/3
  com/1 -> Switch3/1

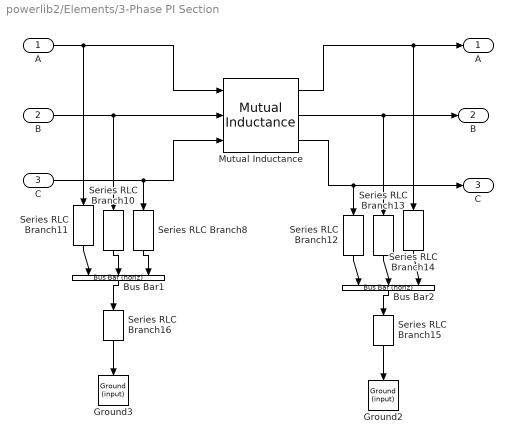
== system powerlib2/Elements/3-Phase PI Section ==
  A : Inport  Port=1  LatchInput=off
  B : Inport  Port=2  LatchInput=off
  C : Inport  Port=3  LatchInput=off
  Bus Bar1 : powerlib2/Connectors/Bus Bar (horiz)  Tag=PoWeRsYsTeMbLoCk  Orientation=down  entrees=3  sorties=1  PSBOutputType=1111111111111111111111111111111111111111111111111111111111111111111111111
  Bus Bar2 : powerlib2/Connectors/Bus Bar (horiz)  Tag=PoWeRsYsTeMbLoCk  Orientation=down  entrees=3  sorties=1  PSBOutputType=1111111111111111111111111111111111111111111111111111111111111111111111111
  Ground2 : powerlib2/Connectors/Ground (input)  Tag=PoWeRsYsTeMbLoCk  Orientation=down
  Ground3 : powerlib2/Connectors/Ground (input)  Tag=PoWeRsYsTeMbLoCk  Orientation=down
  Mutual Inductance : powerlib2/Elements/Mutual Inductance  Tag=PoWeRsYsTeMbLoCk  a=[Rs Ls]  b=[Rs Ls]  w3check=on  c=[Rs Ls]  d=[Rm Lm]  mesure=None  PSBOutputType=111
  Series RLC Branch{8,10..14} (6 alike) : powerlib2/Elements/Series RLC Branch  Tag=PoWeRsYsTeMbLoCk  Orientation=down  a=0  b=0  c=Cp  mesure=None  PSBOutputType=1
  Series RLC Branch15 : powerlib2/Elements/Series RLC Branch  Tag=PoWeRsYsTeMbLoCk  Orientation=down  a=0  b=0  c=Cn  mesure=None  PSBOutputType=1
  Series RLC Branch16 : powerlib2/Elements/Series RLC Branch  Tag=PoWeRsYsTeMbLoCk  Orientation=down  a=0  b=0  c=Cn  mesure=None  PSBOutputType=1
  "A " : Outport  InitialOutput=0
  "B " : Outport  Port=2  InitialOutput=0
  "C " : Outport  Port=3  InitialOutput=0
  wires:
  Series RLC Branch15/1 -> Ground2/1
  Series RLC Branch12/1 -> Bus Bar2/1
  Series RLC Branch13/1 -> Bus Bar2/2
  Series RLC Branch14/1 -> Bus Bar2/3
  Bus Bar2/1 -> Series RLC Branch15/1
  Series RLC Branch11/1 -> Bus Bar1/1
  Series RLC Branch10/1 -> Bus Bar1/2
  Series RLC Branch8/1 -> Bus Bar1/3
  Bus Bar1/1 -> Series RLC Branch16/1
  Series RLC Branch16/1 -> Ground3/1
  C/1 -> Mutual Inductance/3, Series RLC Branch8/1
  B/1 -> Mutual Inductance/2, Series RLC Branch10/1
  A/1 -> Mutual Inductance/1, Series RLC Branch11/1
  Mutual Inductance/3 -> "C "/1, Series RLC Branch12/1
  Mutual Inductance/2 -> "B "/1, Series RLC Branch13/1
  Mutual Inductance/1 -> "A "/1, Series RLC Branch14/1

== system powerlib2/Elements/3-Phase Transformer 12-terminals ==
  A1+ : Inport  Port=1  LatchInput=off
  A1 : Inport  Port=2  LatchInput=off
  B1+ : Inport  Port=3  LatchInput=off
  B1 : Inport  Port=4  LatchInput=off
  C1+ : Inport  Port=5  LatchInput=off
  C1 : Inport  Port=6  LatchInput=off
  T1 : powerlib2/Elements/Linear Transformer  Tag=PoWeRsYsTeMbLoCk  a=[pnom fnom]  b=[ u1 r1 x1]  c=[u2 r2 x2]  w3check=off  d=[u2 r2 x2]  e=rxm  mesure=None  PSBOutputType=1111
  T2 : powerlib2/Elements/Linear Transformer  Tag=PoWeRsYsTeMbLoCk  a=[pnom fnom]  b=[ u1 r1 x1]  c=[u2 r2 x2]  w3check=off  d=[u2 r2 x2]  e=rxm  mesure=None  PSBOutputType=1111
  T3 : powerlib2/Elements/Linear Transformer  Tag=PoWeRsYsTeMbLoCk  a=[pnom fnom]  b=[ u1 r1 x1]  c=[u2 r2 x2]  w3check=off  d=[u2 r2 x2]  e=rxm  mesure=None  PSBOutputType=1111
  A2+ : Outport  InitialOutput=0
  "A2 " : Outport  Port=2  InitialOutput=0
  B2+ : Outport  Port=3  InitialOutput=0
  B2 : Outport  Port=4  InitialOutput=0
  C2+ : Outport  Port=5  InitialOutput=0
  C2 : Outport  Port=6  InitialOutput=0
  wires:
  T1/2 -> "A2 "/1
  A1+/1 -> T1/1
  A1/1 -> T1/2
  B1+/1 -> T2/1
  B1/1 -> T2/2
  C1+/1 -> T3/1
  C1/1 -> T3/2
  T1/1 -> A2+/1
  T2/1 -> B2+/1
  T2/2 -> B2/1
  T3/1 -> C2+/1
  T3/2 -> C2/1

== system powerlib2/Elements/Breaker ==
  1 : Inport  Port=1  LatchInput=off
  c : Inport  Port=2  LatchInput=off
  C4 : Constant  Value=com
  Constant1 : Constant  Value=NaN
  Data Type  Conversion : DataTypeConversion  OutDataTypeMode=double  SaturateOnIntegerOverflow=on  RndMeth=Zero
  Switch3 : Switch  Threshold=0.5  InputSameDT=on
  Terminator : Terminator
  Timer : powerlib_extras/Control  Blocks/Timer  t=times  e=switchings
  2 : Outport  InitialOutput=0
  tag scope: BreakerGotoTag=global
  wires:
  1/1 -> Terminator/1
  Constant1/1 -> 2/1
  Switch3/1 -> [BreakerGotoTag]
  C4/1 -> Switch3/2
  Timer/1 -> Switch3/3
  c/1 -> Data Type  Conversion/1
  Data Type  Conversion/1 -> Switch3/1

== system powerlib2/Elements/Distributed Parameters Line ==
  1 : Inport  Port=1  LatchInput=off
  2 : Inport  Port=2  LatchInput=off
  3 : Inport  Port=3  LatchInput=off
  g1 : Constant
  g2 : Constant
  g3 : Constant
  t1 : Terminator
  t2 : Terminator
  t3 : Terminator
  " 1" : Outport  InitialOutput=0
  " 2" : Outport  Port=2  InitialOutput=0
  " 3" : Outport  Port=3  InitialOutput=0
  wires:
  g1/1 -> " 1"/1
  1/1 -> t1/1
  2/1 -> t2/1
  g2/1 -> " 2"/1
  3/1 -> t3/1
  g3/1 -> " 3"/1

== system powerlib2/Elements/Linear Transformer ==
  in_1 : Inport  Port=1  LatchInput=off
  in_2 : Inport  Port=2  LatchInput=off
  Constant1 : Constant  Value=NaN
  Constant2 : Constant  Value=NaN
  Constant3 : Constant
  Constant4 : Constant
  Terminator : Terminator
  Terminator1 : Terminator
  out_1 : Outport  InitialOutput=0
  out_2 : Outport  Port=2  InitialOutput=0
  out_3 : Outport  Port=3
  out_4 : Outport  Port=4
  wires:
  in_1/1 -> Terminator/1
  in_2/1 -> Terminator1/1
  Constant1/1 -> out_1/1
  Constant2/1 -> out_2/1
  Constant3/1 -> out_3/1
  Constant4/1 -> out_4/1

== system powerlib2/Elements/Mutual Inductance ==
  In_1 : Inport  Port=1  LatchInput=off
  In_2 : Inport  Port=2  LatchInput=off
  in_3 : Inport  Port=3  LatchInput=off
  Constant1 : Constant  Value=NaN
  Constant2 : Constant  Value=NaN
  Constant3 : Constant
  Terminator : Terminator
  Terminator1 : Terminator
  Terminator3 : Terminator
  Outport : Outport  InitialOutput=0
  Outport1 : Outport  Port=2  InitialOutput=0
  out_3 : Outport  Port=3
  wires:
  In_1/1 -> Terminator/1
  In_2/1 -> Terminator1/1
  Constant1/1 -> Outport/1
  Constant2/1 -> Outport1/1
  in_3/1 -> Terminator3/1
  Constant3/1 -> out_3/1

== system powerlib2/Elements/PI Section Line ==
  in : Inport  Port=1  LatchInput=off
  Constant1 : Constant  Value=NaN
  Terminator : Terminator
  out : Outport  InitialOutput=0
  wires:
  in/1 -> Terminator/1
  Constant1/1 -> out/1

== system powerlib2/Elements/Parallel RLC Branch ==
  In_1 : Inport  Port=1  LatchInput=off
  Constant : Constant  Value=NaN
  Terminator : Terminator
  Outport : Outport  InitialOutput=0
  wires:
  In_1/1 -> Terminator/1
  Constant/1 -> Outport/1

== system powerlib2/Elements/Parallel RLC Load ==
  In_1 : Inport  Port=1  LatchInput=off
  Constant : Constant  Value=NaN
  Terminator : Terminator
  Outport : Outport  InitialOutput=0
  wires:
  In_1/1 -> Terminator/1
  Constant/1 -> Outport/1

== system powerlib2/Elements/Saturable Transformer ==
  in_1 : Inport  Port=1  LatchInput=off
  in_2 : Inport  Port=2  LatchInput=off
  Constant1 : Constant  Value=NaN
  Constant2 : Constant  Value=NaN
  Constant3 : Constant
  Constant4 : Constant
  Terminator : Terminator
  Terminator1 : Terminator
  out_1 : Outport  InitialOutput=0
  out_2 : Outport  Port=2  InitialOutput=0
  out_3 : Outport  Port=3
  out_4 : Outport  Port=4
  wires:
  in_1/1 -> Terminator/1
  in_2/1 -> Terminator1/1
  Constant1/1 -> out_1/1
  Constant2/1 -> out_2/1
  Constant3/1 -> out_3/1
  Constant4/1 -> out_4/1

== system powerlib2/Elements/Series RLC Branch ==
  In_1 : Inport  Port=1  LatchInput=off
  Constant : Constant  Value=NaN
  Terminator : Terminator
  Outport : Outport  InitialOutput=0
  wires:
  In_1/1 -> Terminator/1
  Constant/1 -> Outport/1

== system powerlib2/Elements/Series RLC Load ==
  In_1 : Inport  Port=1  LatchInput=off
  Constant : Constant  Value=NaN
  Terminator : Terminator
  Outport : Outport  InitialOutput=0
  wires:
  In_1/1 -> Terminator/1
  Constant/1 -> Outport/1

== system powerlib2/Elements/Surge Arrester ==
  In_1 : Inport  Port=1  LatchInput=off
  Constant1 : Constant  Value=NaN
  Terminator : Terminator
  Outport : Outport  InitialOutput=0
  wires:
  In_1/1 -> Terminator/1
  Constant1/1 -> Outport/1

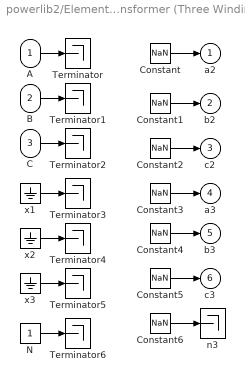
== system powerlib2/Elements/Three-Phase Transformer (Three Windings) ==
  A : Inport  Port=1  LatchInput=off
  B : Inport  Port=2  LatchInput=off
  C : Inport  Port=3  LatchInput=off
  Constant{,1..6} (7 alike) : Constant  Value=NaN
  N : Constant
  Terminator{,1..6} (7 alike) : Terminator
  n3 : Terminator
  x1 : Ground
  x2 : Ground
  x3 : Ground
  a2 : Outport  InitialOutput=0
  b2 : Outport  Port=2  InitialOutput=0
  c2 : Outport  Port=3  InitialOutput=0
  a3 : Outport  Port=4
  b3 : Outport  Port=5
  c3 : Outport  Port=6
  wires:
  Constant6/1 -> n3/1
  N/1 -> Terminator6/1
  A/1 -> Terminator/1
  B/1 -> Terminator1/1
  C/1 -> Terminator2/1
  x1/1 -> Terminator3/1
  x2/1 -> Terminator4/1
  x3/1 -> Terminator5/1
  Constant/1 -> a2/1
  Constant1/1 -> b2/1
  Constant2/1 -> c2/1
  Constant3/1 -> a3/1
  Constant4/1 -> b3/1
  Constant5/1 -> c3/1

== system powerlib2/Elements/Three-phase Transformer (Two Windings) ==
  A : Inport  Port=1  LatchInput=off
  B : Inport  Port=2  LatchInput=off
  C : Inport  Port=3  LatchInput=off
  N : Inport  Port=4  LatchInput=off
  Constant{,1..3} (4 alike) : Constant  Value=NaN
  Terminator{,1..3} (4 alike) : Terminator
  a : Outport  InitialOutput=0
  b : Outport  Port=2  InitialOutput=0
  c : Outport  Port=3  InitialOutput=0
  n : Outport  Port=4
  wires:
  Constant3/1 -> n/1
  N/1 -> Terminator3/1
  Constant/1 -> a/1
  A/1 -> Terminator/1
  B/1 -> Terminator1/1
  C/1 -> Terminator2/1
  Constant1/1 -> b/1
  Constant2/1 -> c/1

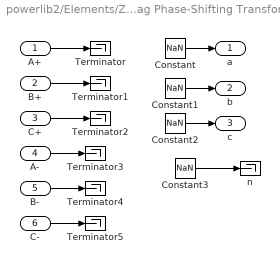
== system powerlib2/Elements/Zigzag Phase-Shifting Transformer ==
  A+ : Inport  Port=1  LatchInput=off
  B+ : Inport  Port=2  LatchInput=off
  C+ : Inport  Port=3  LatchInput=off
  A- : Inport  Port=4  LatchInput=off
  B- : Inport  Port=5  LatchInput=off
  C- : Inport  Port=6  LatchInput=off
  Constant{,1..3} (4 alike) : Constant  Value=NaN
  Terminator{,1..5} (6 alike) : Terminator
  n : Terminator
  a : Outport  InitialOutput=0
  b : Outport  Port=2  InitialOutput=0
  c : Outport  Port=3  InitialOutput=0
  wires:
  Constant3/1 -> n/1
  A+/1 -> Terminator/1
  B+/1 -> Terminator1/1
  C+/1 -> Terminator2/1
  A-/1 -> Terminator3/1
  B-/1 -> Terminator4/1
  C-/1 -> Terminator5/1
  Constant/1 -> a/1
  Constant1/1 -> b/1
  Constant2/1 -> c/1

== system powerlib2/Machines/Asynchronous Machine SI Units ==
  "A " : Inport  Port=1  LatchInput=off
  "B " : Inport  Port=2  LatchInput=off
  "C " : Inport  Port=3  LatchInput=off
  Tm : Inport  Port=4  LatchInput=off
  Constant1 : Constant
  Constant2 : Constant
  Terminator : Terminator
  Terminator1 : Terminator
  Terminator2 : Terminator
  a : Outport
  b : Outport  Port=2
  c : Outport  Port=3
  m : Outport  Port=4  InitialOutput=0
  tag scope: tp200459=global
  wires:
  Tm/1 -> [tp200459]
  [tp200466] -> m/1, a/1
  "A "/1 -> Terminator/1
  "B "/1 -> Terminator1/1
  "C "/1 -> Terminator2/1
  Constant1/1 -> b/1
  Constant2/1 -> c/1

== system powerlib2/Machines/Asynchronous Machine pu Units ==
  "A " : Inport  Port=1  LatchInput=off
  "B " : Inport  Port=2  LatchInput=off
  "C " : Inport  Port=3  LatchInput=off
  Tm : Inport  Port=4  LatchInput=off
  Constant1 : Constant
  Constant2 : Constant
  Terminator : Terminator
  Terminator1 : Terminator
  Terminator2 : Terminator
  a : Outport
  b : Outport  Port=2
  c : Outport  Port=3
  m : Outport  Port=4  InitialOutput=0
  tag scope: tp200471=global
  wires:
  [tp200476] -> m/1, a/1
  "A "/1 -> Terminator/1
  "B "/1 -> Terminator1/1
  "C "/1 -> Terminator2/1
  Constant1/1 -> b/1
  Constant2/1 -> c/1
  Tm/1 -> [tp200471]
